simulink model "SingleTrack"  (Simulink 7.9)
settings: Solver=ode45  SolverMode=SingleTasking  StartTime=0.0  StopTime=inf  FixedStep=0.001  RelTol=1e-3
PreLoadFcn:
  | SingleTrack_params
undefined symbols (not defined in the file or in its folder): Car_Bdy1_mass, Car_Steering_i, Car_Whl_Radius, Car_WhlBaseF, Car_WhlBaseR, mEngineMax, PT_DL_iDiff, PT_GearBox_iForwardGears
libraries: CarMaker4SL x5
(part 4 of 4)

== system SingleTrack/CarMaker/Vehicle/User Vehicle (CM4SL)/CarAndTrailer/single-track mass point model/yaw/side forces ==
  vYaw : Inport
  beta : Inport  Port=2
  v : Inport  Port=3
  StWhlAngle : Inport  Port=4
  " " : Product  SaturateOnIntegerOverflow=on  InputSameDT=on  OutDataTypeStr=Inherit: Same as first input
  "  " : Product  SaturateOnIntegerOverflow=on  InputSameDT=on  OutDataTypeStr=Inherit: Same as first input
  "            " : Product  SaturateOnIntegerOverflow=on  InputSameDT=on  OutDataTypeStr=Inherit: Same as first input
  "S_R * l_R " : Product  SaturateOnIntegerOverflow=on  InputSameDT=on  OutDataTypeStr=Inherit: Same as first input
  "S_V * l_V " : Product  SaturateOnIntegerOverflow=on  InputSameDT=on  OutDataTypeStr=Inherit: Same as first input
  Subsystem : Subsystem
  Sum : Sum  SaturateOnIntegerOverflow=on  InputSameDT=on  OutDataTypeStr=Inherit: Same as first input
  Sum1 : Sum  Inputs=-+  SaturateOnIntegerOverflow=on  InputSameDT=on  OutDataTypeStr=Inherit: Same as first input
  Sum4 : Sum  Inputs=+-  SaturateOnIntegerOverflow=on  InputSameDT=on  OutDataTypeStr=Inherit: Same as first input
  c_alphaR : Gain  Gain=50000  SaturateOnIntegerOverflow=on  OutDataTypeStr=Inherit: Same as input  ParamDataTypeStr=Inherit: Same as input
  front wheel steering lock angle : Subsystem
  l__F : Constant  Value=Car_WhlBaseF
  l__R : Constant  Value=-Car_WhlBaseR
  S_F * l_F : Outport
  S_R * l_R : Outport  Port=2
  S_V : Outport  Port=3
  S_R : Outport  Port=4
  alpha_F : Outport  Port=5
  alpha_R : Outport  Port=6
  wires:
  front wheel steering lock angle/1(c_alphaF) -> "            "/1
  StWhlAngle/1 -> front wheel steering lock angle/1(StWhlAngle)
  "S_R * l_R "/1 -> S_R * l_R/1
  Sum4/1 -> alpha_F/1, "            "/2
  front wheel steering lock angle/2(delta_F) -> Sum4/1
  Sum/1 -> front wheel steering lock angle/2(beta + l_F * vYaw / v), Sum4/2
  v/1 -> Subsystem/1(v)
  vYaw/1 -> Subsystem/2(vYaw)
  "S_V * l_V "/1 -> S_F * l_F/1
  "            "/1 -> S_V/1, "S_V * l_V "/1
  c_alphaR/1 -> S_R/1, "S_R * l_R "/1
  Sum1/1 -> alpha_R/1, c_alphaR/1
  "  "/1 -> Sum/2
  " "/1 -> Sum1/2
  l__R/1 -> "S_R * l_R "/2, " "/2
  Subsystem/1(vYaw/v) -> "  "/2, " "/1
  l__F/1 -> "S_V * l_V "/2, "  "/1
  beta/1 -> Sum/1, Sum1/1

== system SingleTrack/CarMaker/Vehicle/User Vehicle (CM4SL)/CarAndTrailer/single-track mass point model/yaw/sideslip angle ==
  vYaw : Inport
  m : Inport  Port=2
  v_dot : Inport  Port=3
  v : Inport  Port=4
  S : Inport  Port=5
  " " : Product  Inputs=*/  SaturateOnIntegerOverflow=on  InputSameDT=on  OutDataTypeStr=Inherit: Same as first input
  "  " : Product  SaturateOnIntegerOverflow=on  InputSameDT=on  OutDataTypeStr=Inherit: Same as first input
  Subsystem : Subsystem
  Sum2 : Sum  Inputs=+-  SaturateOnIntegerOverflow=on  InputSameDT=on  OutDataTypeStr=Inherit: Same as first input
  beta_dot * dt : Integrator  ExternalReset=level
  beta_dot : Outport
  beta : Outport  Port=2
  wires:
  v/1 -> Subsystem/2(v)
  Subsystem/1(Out1) -> beta_dot/1, beta_dot * dt/1
  vYaw/1 -> Subsystem/1(vYaw)
  Sum2/1 -> Subsystem/3(In3)
  "  "/1 -> Sum2/2
  m/1 -> " "/2
  v_dot/1 -> "  "/1
  " "/1 -> Sum2/1
  S/1 -> " "/1
  beta_dot * dt/1 -> "  "/2, beta/1
  [TRStart] -> beta_dot * dt/2

== system SingleTrack/CarMaker/Vehicle/User Vehicle (CM4SL)/CarAndTrailer/PowerTrainUpd/Set OperationState/If Action Subsystem/If Action Subsystem ==
  In1 : Inport
  Action Port : ActionPort  ActionType=then
  Out1 : Outport
  wires:
  In1/1 -> Out1/1

== system SingleTrack/CarMaker/Vehicle/User Vehicle (CM4SL)/CarAndTrailer/PowerTrainUpd/Set OperationState/If Action Subsystem/If Action Subsystem1 ==
  In1 : Inport
  Action Port : ActionPort  ActionType=else
  Out1 : Outport
  wires:
  In1/1 -> Out1/1

== system SingleTrack/CarMaker/Vehicle/User Vehicle (CM4SL)/CarAndTrailer/single-track mass point model/yaw/Vehicle Initial Cfg/CreateBus Vhcl.Cfg ==
  In1 : Inport
  Bus Creator : BusCreator  Inputs=13
  Demux : Demux  Outputs=13
  Out1 : Outport
  wires:
  Demux/13 -> Bus Creator/13  "Vhcl Cfg Whl_rotv RR"
  Bus Creator/1 -> Out1/1
  In1/1 -> Demux/1
  Demux/12 -> Bus Creator/12  "Vhcl Cfg Whl_rotv RL"
  Demux/11 -> Bus Creator/11  "Vhcl Cfg Whl_rotv FR"
  Demux/10 -> Bus Creator/10  "Vhcl Cfg Whl_rotv FL"
  Demux/9 -> Bus Creator/9  "SimCore Trailer nTrailers"
  Demux/8 -> Bus Creator/8  "Vhcl Cfg GearBox_rotv_out"
  Demux/7 -> Bus Creator/7  "Vhcl Cfg Engine_rotv"
  Demux/6 -> Bus Creator/6  "Vhcl Cfg Pitch"
  Demux/5 -> Bus Creator/5  "Vhcl Cfg Yaw"
  Demux/4 -> Bus Creator/4  "Vhcl Cfg Roll"
  Demux/2 -> Bus Creator/2  "Vhcl Cfg Fr1_Pos y"
  Demux/1 -> Bus Creator/1  "Vhcl Cfg Fr1_Pos x"
  Demux/3 -> Bus Creator/3  "Vhcl Cfg Fr1_Pos z"

== system SingleTrack/CarMaker/Vehicle/User Vehicle (CM4SL)/CarAndTrailer/single-track mass point model/yaw/side forces/Subsystem ==
  v : Inport
  vYaw : Inport  Port=2
  If : If  IfExpression=u1 > 0.1 | u1 < -0.1
  If Action Subsystem : Subsystem  TreatAsAtomicUnit=on
  If Action Subsystem1 : Subsystem  TreatAsAtomicUnit=on
  Merge : Merge  InitialOutput=0
  vYaw/v : Outport
  wires:
  v/1 -> If Action Subsystem/1(v), If/1
  vYaw/1 -> If Action Subsystem/2(vYaw)
  If/1 -> If Action Subsystem/Action
  If/2 -> If Action Subsystem1/Action
  Merge/1 -> vYaw/v/1
  If Action Subsystem/1(Out1) -> Merge/1
  If Action Subsystem1/1(Out1) -> Merge/2

== system SingleTrack/CarMaker/Vehicle/User Vehicle (CM4SL)/CarAndTrailer/single-track mass point model/yaw/side forces/front wheel steering lock angle ==
  StWhlAngle : Inport
  beta + l_F * vYaw / v : Inport  Port=2
  "   " : Product  SaturateOnIntegerOverflow=on  InputSameDT=on  OutDataTypeStr=Inherit: Same as first input
  "     " : Constant
  "      " : Product  Inputs=*/  SaturateOnIntegerOverflow=on  InputSameDT=on  OutDataTypeStr=Inherit: Same as first input
  "       " : Product  Inputs=*/*  SaturateOnIntegerOverflow=on  InputSameDT=on  OutDataTypeStr=Inherit: Same as first input
  1/ i_S : Gain  Gain=1/Car_Steering_i  SaturateOnIntegerOverflow=on  OutDataTypeStr=Inherit: Same as input  ParamDataTypeStr=Inherit: Same as input
  C_S : Constant  Value=10000
  Sum2 : Sum  SaturateOnIntegerOverflow=on  InputSameDT=on  OutDataTypeStr=Inherit: Same as first input
  Sum3 : Sum  SaturateOnIntegerOverflow=on  InputSameDT=on  OutDataTypeStr=Inherit: Same as first input
  "c_alphaF " : Constant  Value=50000
  n_F : Constant  Value=0.06
  c_alphaF : Outport
  delta_F : Outport  Port=2
  wires:
  "      "/1 -> delta_F/1
  "c_alphaF "/1 -> "       "/1, c_alphaF/1
  n_F/1 -> "       "/3
  C_S/1 -> "       "/2
  Sum2/1 -> "      "/1
  Sum3/1 -> "      "/2
  "     "/1 -> Sum3/1
  1/ i_S/1 -> Sum2/1
  "   "/1 -> Sum2/2
  StWhlAngle/1 -> 1/ i_S/1
  "       "/1 -> "   "/1, Sum3/2
  beta + l_F * vYaw / v/1 -> "   "/2

== system SingleTrack/CarMaker/Vehicle/User Vehicle (CM4SL)/CarAndTrailer/single-track mass point model/yaw/sideslip angle/Subsystem ==
  vYaw : Inport
  v : Inport  Port=2
  In3 : Inport  Port=3
  If : If  IfExpression=u1 > 0.1 | u1 < -0.1
  If Action Subsystem : Subsystem  TreatAsAtomicUnit=on
  If Action Subsystem1 : Subsystem  TreatAsAtomicUnit=on
  Merge : Merge
  Sum1 : Sum  Inputs=-+  SaturateOnIntegerOverflow=on  InputSameDT=on  OutDataTypeStr=Inherit: Same as first input
  Out1 : Outport
  wires:
  vYaw/1 -> Sum1/1
  v/1 -> If Action Subsystem/1(v), If/1
  Sum1/1 -> Out1/1
  If Action Subsystem/1(Out1) -> Merge/1
  If Action Subsystem1/1(Out1) -> Merge/2
  Merge/1 -> Sum1/2
  If/2 -> If Action Subsystem1/Action
  In3/1 -> If Action Subsystem/2(In3)
  If/1 -> If Action Subsystem/Action

== system SingleTrack/CarMaker/Vehicle/User Vehicle (CM4SL)/CarAndTrailer/single-track mass point model/yaw/side forces/Subsystem/If Action Subsystem ==
  v : Inport
  vYaw : Inport  Port=2
  Action Port : ActionPort  ActionType=then
  vYaw / v : Product  Inputs=/*  SaturateOnIntegerOverflow=on  InputSameDT=on  OutDataTypeStr=Inherit: Same as first input
  Out1 : Outport  InitialOutput=0
  wires:
  v/1 -> vYaw / v/1
  vYaw/1 -> vYaw / v/2
  vYaw / v/1 -> Out1/1

== system SingleTrack/CarMaker/Vehicle/User Vehicle (CM4SL)/CarAndTrailer/single-track mass point model/yaw/side forces/Subsystem/If Action Subsystem1 ==
  Action Port : ActionPort  ActionType=else
  Constant : Constant  Value=0
  Out1 : Outport  InitialOutput=0
  wires:
  Constant/1 -> Out1/1

== system SingleTrack/CarMaker/Vehicle/User Vehicle (CM4SL)/CarAndTrailer/single-track mass point model/yaw/sideslip angle/Subsystem/If Action Subsystem ==
  v : Inport
  In3 : Inport  Port=2
  Action Port : ActionPort  ActionType=then
  "    " : Product  Inputs=/*  SaturateOnIntegerOverflow=on  InputSameDT=on  OutDataTypeStr=Inherit: Same as first input
  Out1 : Outport  InitialOutput=0
  wires:
  v/1 -> "    "/1
  In3/1 -> "    "/2
  "    "/1 -> Out1/1

== system SingleTrack/CarMaker/Vehicle/User Vehicle (CM4SL)/CarAndTrailer/single-track mass point model/yaw/sideslip angle/Subsystem/If Action Subsystem1 ==
  Action Port : ActionPort  ActionType=else
  Constant : Constant  Value=0
  Out1 : Outport  InitialOutput=0
  wires:
  Constant/1 -> Out1/1
